simulink model "Second_disconnected"  (R2015b)
settings: Solver=VariableStepAuto  StartTime=0.0  StopTime=6.58  FixedStep=0.02  RelTol=1e-3
values from neighbouring files (symbols this model uses):
  D = 1.7*10^-5    (= 1.7e-05)    [Project3_matlab.m]    (also in backup_connected.m; connected_La_zero.m; connected_current_speed.m; connected_current_speed_La_zero.m)
  Jm = 4.7*10^-5    (= 4.7e-05)    [Project3_matlab.m]    (also in backup_connected.m; connected_La_zero.m; connected_current_speed.m; connected_current_speed_La_zero.m)
  Ke = 7.06*10^-2    (= 0.0706)    [Project3_matlab.m]    (also in backup_connected.m; connected_La_zero.m; connected_current_speed.m; connected_current_speed_La_zero.m)
  Kt = 7.06*10^-2    (= 0.0706)    [Project3_matlab.m]    (also in backup_connected.m; connected_La_zero.m; connected_current_speed.m; connected_current_speed_La_zero.m)
  La = 0.87*10^-3    (= 0.00087)    [Project3_matlab.m]    (also in backup_connected.m; connected_La_zero.m = 0; connected_current_speed.m; connected_current_speed_La_zero.m = 0)
  Ra = 0.59    [Project3_matlab.m]    (also in backup_connected.m; connected_La_zero.m; connected_current_speed.m; connected_current_speed_La_zero.m)
settings Model: Creator=guilh_000  LastModifiedBy=guilh_000

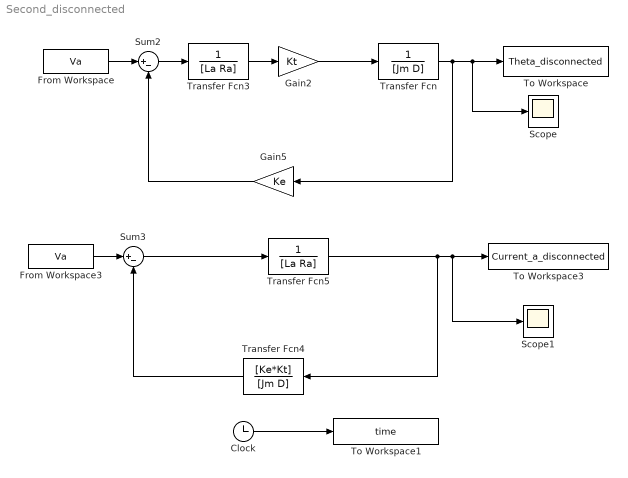
== system Second_disconnected ==
  Clock : Clock
  From Workspace : FromWorkspace  VariableName=Va
  From Workspace3 : FromWorkspace  VariableName=Va
  Gain2 : Gain  Gain=Kt
  Gain5 : Gain  Gain=Ke
  Scope : Scope
  Scope1 : Scope
  Sum2 : Sum  Inputs=|+-
  Sum3 : Sum  Inputs=|+-
  To Workspace : ToWorkspace  VariableName=Theta_disconnected  SampleTime=-1
  To Workspace1 : ToWorkspace  VariableName=time  SampleTime=-1
  To Workspace3 : ToWorkspace  VariableName=Current_a_disconnected  SampleTime=-1
  Transfer Fcn : TransferFcn  Denominator=[Jm D]
  Transfer Fcn3 : TransferFcn  Denominator=[La Ra]
  Transfer Fcn4 : TransferFcn  Numerator=[Ke*Kt]  Denominator=[Jm D]
  Transfer Fcn5 : TransferFcn  Denominator=[La Ra]
  wires:
  Sum2/1 -> Transfer Fcn3/1
  Transfer Fcn3/1 -> Gain2/1
  Gain2/1 -> Transfer Fcn/1
  Transfer Fcn/1 -> Gain5/1, Scope/1, To Workspace/1
  Gain5/1 -> Sum2/2
  From Workspace/1 -> Sum2/1
  Sum3/1 -> Transfer Fcn5/1
  Transfer Fcn5/1 -> Transfer Fcn4/1, Scope1/1, To Workspace3/1
  Transfer Fcn4/1 -> Sum3/2
  From Workspace3/1 -> Sum3/1
  Clock/1 -> To Workspace1/1
